simulink model "sampleModel372"  (R2021b)
settings: Solver=VariableStepAuto  StartTime=0.0  StopTime=10.0  RelTol=1e-3
undefined symbols (not defined in the file or in its folder): DiscIntNeverNeededParam, Newton, Raphson
libraries: simulink x10, slpidlib x1
settings Model: Creator=user  LastModifiedBy=user

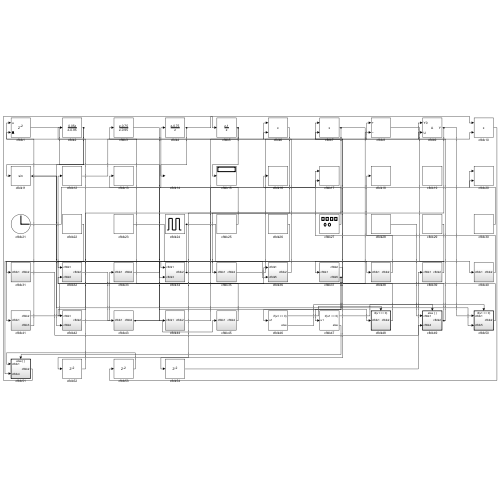
[thumbnail: Simulink's stored preview of the top-level diagram]
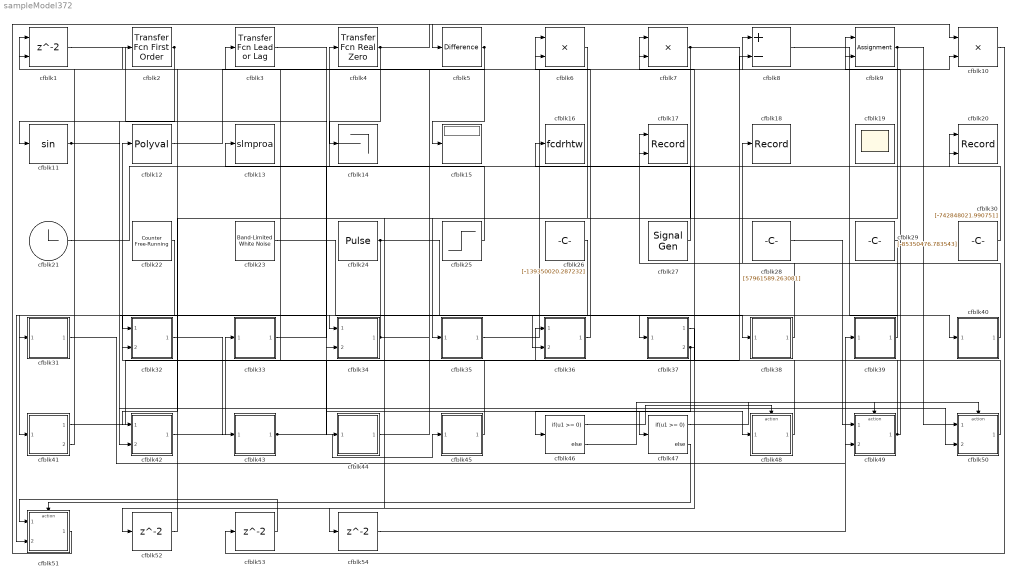
== system sampleModel372 ==
  cfblk1 : Delay  ShowEnablePort=on  SampleTime=1
      settings: InputPortMap=u0,e6
  cfblk10 : Product
  cfblk11 : Trigonometry
  cfblk12 : Polyval  Coefs=[ +2.081618890e-019, -1.441693666e-014, +4.719686976e-010, -8.536869453e-006, +1.621573104e-001, -8.087801117e+001 ]
  cfblk13 : ToWorkspace  VariableName=slmproa  SaveFormat=Timeseries  SampleTime=-1
  cfblk14 : Terminator
  cfblk15 : Display
  cfblk16 : ToWorkspace  VariableName=fcdrhtw  SaveFormat=Timeseries  SampleTime=-1
  cfblk17 : Record  FileSettingsInternal="{\"entries\":[{\"content\":{\"excelSettings\":{\"content\":{},\"type\":\"Streamout.ExcelSettings\"}},\"type\":\"Streamout.FileSettingStorage\",\"uuid\":\"b72ebad9-7056-485c-ac51-affa3a1e9353\"}],\"packageUris\":[\"http://schema.mathworks.com/mf0/streamout_blocks/R2020a\"],\"version\":\"1.0\"}"  Layout=[1 1]  SignalsInternal="{\"entries\":[{\"content\":{\"signals\":[{\"content\":{\"blockPath\":[\"sampleModel372/cfblk17\"],\"channel\":[],\"dimensions\":[1],\"domain\":\"sampleModel372/cfblk17\",\"lineColor\":\"#a2142f\",\"plots\":[1],\"port\":1,\"sid\":[\"\"],\"signalID\":15476,\"signalName\":\"cfblk44\"},\"type\":\"RecordBlkView.Signal\",\"uuid\":\"5dfffff1-d32b-4c9b-bc7a-56c91156797a\"},{\"content\":{\"blockPath\":[\"sampleModel372/cfblk17\"],\"channel\":[],\"dimensions\":[1],\"domain\":\"sampleModel372/cfblk17\",\"lineColor\":\"#139fff\",\"plots\":[1],\"port\":2,\"sid\":[\"\"],\"signalID\":15480,\"signalName\":\"cfblk38\"},\"type\":\"RecordBlkView.Signal\",\"uuid\":\"1c828c9b-06c4-4cee-a281-7d6f80fdea4d\"}]},\"type\":\"RecordBlkView.InputSignals\",\"uuid\":\"3665fb33-e0ad-4ba6-b3fb-c5c2c897735a\"}],\"packageUris\":[\"http://schema.mathworks.com/mf0/streamout_blocks/R2020a\"],\"version\":\"1.0\"}"  VisualizationBindings="{\"xyplotplugin\":{\"info\":[{\"series\":[{\"bindingParametersList\":[{\"parameter\":\"X-Axis\",\"signalID\":15476,\"signalName\":\"cfblk44\"},{\"parameter\":\"Y-Axis\",\"signalID\":15480,\"signalName\":\"cfblk38\"}],\"seriesID\":33208}],\"subplotID\":1}]}}"  CompatibilityTag=XY
  cfblk18 : Record  FileSettingsInternal="{\"entries\":[{\"content\":{\"excelSettings\":{\"content\":{},\"type\":\"Streamout.ExcelSettings\"}},\"type\":\"Streamout.FileSettingStorage\",\"uuid\":\"4903c734-b3f9-41ef-b0a2-174ee0824f37\"}],\"packageUris\":[\"http://schema.mathworks.com/mf0/streamout_blocks/R2020a\"],\"version\":\"1.0\"}"  SignalsInternal="{\"entries\":[{\"content\":{\"signals\":[{\"content\":{\"blockPath\":[\"sampleModel372/cfblk18\"],\"channel\":[],\"dimensions\":[1],\"domain\":\"sampleModel372/cfblk18\",\"lineColor\":\"#139fff\",\"plots\":[1],\"port\":1,\"sid\":[\"\"],\"signalID\":15484,\"signalName\":\"cfblk40\"},\"type\":\"RecordBlkView.Signal\",\"uuid\":\"409c68b6-5e7e-4f45-9345-40e6c37d40ec\"}]},\"type\":\"RecordBlkView.InputSignals\",\"uuid\":\"2f5d807f-9e3a-4e8f-8a79-911276b8b2d7\"}],\"packageUris\":[\"http://schema.mathworks.com/mf0/streamout_blocks/R2020a\"],\"version\":\"1.0\"}"  VisualizationBindings="{\"sparklinesplugin\":{\"info\":[{\"bindingParametersList\":[],\"subplotID\":1}]}}"
  cfblk19 : Scope
      settings: Floating=on
  cfblk2 : simulink/Discrete/Transfer Fcn First Order  PoleZ=0.95  ICPrevOutput=0.0  DoSatur=off
  cfblk20 : Record  FileSettingsInternal="{\"entries\":[{\"content\":{\"excelSettings\":{\"content\":{},\"type\":\"Streamout.ExcelSettings\"}},\"type\":\"Streamout.FileSettingStorage\",\"uuid\":\"bf4a5471-e929-4e71-bb99-9183bb1d84e0\"}],\"packageUris\":[\"http://schema.mathworks.com/mf0/streamout_blocks/R2020a\"],\"version\":\"1.0\"}"  Layout=[1 1]  SignalsInternal="{\"entries\":[{\"content\":{\"signals\":[{\"content\":{\"blockPath\":[\"sampleModel372/cfblk20\"],\"channel\":[],\"dimensions\":[1],\"domain\":\"sampleModel372/cfblk20\",\"lineColor\":\"#a2142f\",\"plots\":[1],\"port\":1,\"sid\":[\"\"],\"signalID\":15488,\"signalName\":\"cfblk33\"},\"type\":\"RecordBlkView.Signal\",\"uuid\":\"8512df04-6121-435b-9967-1d101e83269f\"},{\"content\":{\"blockPath\":[\"sampleModel372/cfblk20\"],\"channel\":[],\"dimensions\":[1],\"domain\":\"sampleModel372/cfblk20\",\"lineColor\":\"#139fff\",\"plots\":[1],\"port\":2,\"sid\":[\"\"],\"signalID\":15492,\"signalName\":\"cfblk30\"},\"type\":\"RecordBlkView.Signal\",\"uuid\":\"2aaa770d-525c-4c22-91f0-bfea3dd1c119\"}]},\"type\":\"RecordBlkView.InputSignals\",\"uuid\":\"b4e04a43-241c-40c6-8415-553e41d5351d\"}],\"packageUris\":[\"http://schema.mathworks.com/mf0/streamout_blocks/R2020a\"],\"version\":\"1.0\"}"  VisualizationBindings="{\"xyplotplugin\":{\"info\":[{\"series\":[{\"bindingParametersList\":[{\"parameter\":\"X-Axis\",\"signalID\":15488,\"signalName\":\"cfblk33\"},{\"parameter\":\"Y-Axis\",\"signalID\":15492,\"signalName\":\"cfblk30\"}],\"seriesID\":31222}],\"subplotID\":1}]}}"  CompatibilityTag=XY
  cfblk21 : Clock
  cfblk22 : simulink/Sources/Counter Free-Running  NumBits=[31.000000]  tsamp=-1
  cfblk23 : simulink/Sources/Band-Limited White Noise  Cov=[6149014609.811703]  Ts=0.1  seed=[2691800699.000000]
  cfblk24 : DiscretePulseGenerator  PulseType=Time based  Amplitude=[651098866.596543]  Period=[5211290.232713]  PulseWidth=5  PhaseDelay=[5.000000]
  cfblk25 : Step  Time=[32.000000]  Before=[-358467154.042758]  After=[548541878.025109]  SampleTime=0
  cfblk26 : Constant  Value=[-139350020.287232]  SampleTime=1
  cfblk27 : SignalGenerator  WaveForm=sawtooth  Amplitude=[-88090145.710845]
  cfblk28 : Constant  Value=[57961589.263081]  SampleTime=1
  cfblk29 : Constant  Value=[-85350476.783543]  SampleTime=1
  cfblk3 : simulink/Discrete/Transfer Fcn Lead or Lag  PoleZ=0.95  ZeroZ=0.75  ICPrevOutput=0.0  ICPrevInput=0.0  DoSatur=off
      settings: SourceProductBaseCode=SL
  cfblk30 : Constant  Value=[-742848021.990751]  SampleTime=1
  cfblk31 : Subsystem
  cfblk32 : Subsystem
  cfblk33 : Subsystem
  cfblk34 : Subsystem
  cfblk35 : Subsystem
  cfblk36 : Subsystem
  cfblk37 : Subsystem
  cfblk38 : Subsystem
  cfblk39 : Subsystem
  cfblk4 : simulink/Discrete/Transfer Fcn Real Zero  ZeroZ=0.75  ICPrevInput=0.0  DoSatur=off
      settings: SourceProductBaseCode=SL
  cfblk40 : Subsystem
  cfblk41 : Subsystem
  cfblk42 : Subsystem
  cfblk43 : Subsystem
  cfblk44 : Subsystem
  cfblk45 : Subsystem
  cfblk46 : If  IfExpression=u1 >= 0  SampleTime=1
  cfblk47 : If  IfExpression=u1 >= 0  SampleTime=1
  cfblk48 : Subsystem  TreatAsAtomicUnit=on
  cfblk49 : Subsystem  TreatAsAtomicUnit=on
  cfblk5 : simulink/Discrete/Difference  ICPrevInput=0.0  OutMin=[]  OutMax=[]  OutDataTypeStr=Inherit: Inherit via back propagation  OutDataType=fixdt(1, 16)  OutScaling=2^-10  DoSatur=off
  cfblk50 : Subsystem  TreatAsAtomicUnit=on
  cfblk51 : Subsystem  TreatAsAtomicUnit=on
  cfblk52 : Delay  SampleTime=1
  cfblk53 : Delay  SampleTime=1
  cfblk54 : Delay  SampleTime=1
  cfblk6 : Product  Inputs=**
  cfblk7 : Product
  cfblk8 : Sum  Inputs=+-
  cfblk9 : Assignment  DiagnosticForDimensions=Warning  IndexOptions=Index vector (dialog)  Indices=1  OutputSizes=1
  wires:
  cfblk9/1 -> cfblk35/1(cfblk1), cfblk50/1(cfblk1)
  cfblk35/1(cfblk2) -> cfblk8/1
  cfblk21/1 -> cfblk4/1
  cfblk5/1 -> cfblk15/1, cfblk1/2
  cfblk25/1 -> cfblk13/1
  cfblk3/1 -> cfblk48/1(cfblk1)
  cfblk43/1(cfblk2) -> cfblk45/1(cfblk1), cfblk36/1(cfblk1)
  cfblk4/1 -> cfblk14/1, cfblk10/1
  cfblk45/1(cfblk2) -> cfblk12/1
  cfblk2/1 -> cfblk11/1, cfblk42/2(cfblk4)
  cfblk31/1(cfblk2) -> cfblk39/1(cfblk1)
  cfblk42/1(cfblk2) -> cfblk33/1(cfblk1)
  cfblk26/1 -> cfblk34/1(cfblk1)
  cfblk51/1(cfblk2) -> cfblk5/1
  cfblk33/1(cfblk2) -> cfblk20/1
  cfblk50/1(cfblk2) -> cfblk3/1
  cfblk29/1 -> cfblk32/1(cfblk1)
  cfblk22/1 -> cfblk41/1(cfblk1)
  cfblk30/1 -> cfblk20/2
  cfblk1/1 -> cfblk44/1(cfblk1)
  cfblk39/1(cfblk2) -> cfblk37/1(cfblk1)
  cfblk28/1 -> cfblk49/1(cfblk1)
  cfblk27/1 -> cfblk16/1
  cfblk12/1 -> cfblk9/1
  cfblk24/1 -> cfblk51/2(cfblk4), cfblk36/2(cfblk5)
  cfblk36/1(cfblk2) -> cfblk6/1
  cfblk44/1(cfblk2) -> cfblk17/1
  cfblk40/1(cfblk2) -> cfblk18/1
  cfblk38/1(cfblk2) -> cfblk17/2
  cfblk8/1 -> cfblk40/1(cfblk1)
  cfblk23/1 -> cfblk38/1(cfblk1)
  cfblk11/1 -> cfblk34/2(cfblk3), cfblk50/2(cfblk5)
  cfblk41/1(cfblk2) -> cfblk8/2
  cfblk37/2(cfblk5) -> cfblk47/1, cfblk7/2, cfblk46/1
  cfblk48/1(cfblk2) -> cfblk7/1
  cfblk32/1(cfblk2) -> cfblk43/1(cfblk1)
  cfblk41/2(cfblk3) -> cfblk1/1
  cfblk49/1(cfblk2) -> cfblk9/2, cfblk32/2(cfblk3)
  cfblk7/1 -> cfblk42/1(cfblk1), cfblk10/2
  cfblk34/1(cfblk2) -> cfblk31/1(cfblk1), cfblk6/2
  cfblk46/1 -> cfblk48/Action
  cfblk46/2 -> cfblk49/Action
  cfblk47/1 -> cfblk50/Action
  cfblk47/2 -> cfblk51/Action
  cfblk37/1(cfblk2) -> cfblk52/1
  cfblk52/1 -> cfblk2/1
  cfblk10/1 -> cfblk53/1
  cfblk53/1 -> cfblk51/1(cfblk1)
  cfblk6/1 -> cfblk54/1
  cfblk54/1 -> cfblk49/2(cfblk4)

== system sampleModel372/cfblk31 ==
  cfblk1 : Inport
  cfblk3 : slpidlib/PID Controller (2DOF)  Controller=PID  Form=Parallel  TimeDomain=Discrete-time  UseExternalTs=off  SampleTime=1  IntegratorMethod=Forward Euler  FilterMethod=Forward Euler  ControllerParametersSource=internal  P=1  I=1  D=0  UseFilter=on  N=100  b=1  c=1  TunerSelectOption=Transfer Function Based (PID Tuner App)  InitialConditionSource=internal  InitialConditionForIntegrator=0  InitialConditionForFilter=0  DifferentiatorICPrevScaledInput=0  ExternalReset=none  TrackingMode=off  Kt=1  LimitOutput=off  SatLimitsSource=internal  UpperSaturationLimit=inf  LowerSaturationLimit=-inf  LinearizeAsGain=off  AntiWindupMode=none  Kb=1  POutMin=[]  POutMax=[]  IOutMin=[]  IOutMax=[]  DOutMin=[]  DOutMax=[]  NOutMin=[]  NOutMax=[]  bOutMin=[]  bOutMax=[]  cOutMin=[]  cOutMax=[]  SumOutMin=[]  SumOutMax=[]  SaturationOutMin=[]  SaturationOutMax=[]  PParamMin=[]  PParamMax=[]  IParamMin=[]  IParamMax=[]  DParamMin=[]  DParamMax=[]  NParamMin=[]  NParamMax=[]  bParamMin=[]  bParamMax=[]  cParamMin=[]  cParamMax=[]  KbParamMin=[]  KbParamMax=[]  KtParamMin=[]  KtParamMax=[]  KbOutMin=[]  KbOutMax=[]  KtOutMin=[]  KtOutMax=[]  IntegratorOutMin=[]  IntegratorOutMax=[]  FilterOutMin=[]  FilterOutMax=[]  SumI1OutMin=[]  SumI1OutMax=[]  SumI2OutMin=[]  SumI2OutMax=[]  SumI3OutMin=[]  SumI3OutMax=[]  SumI4OutMin=[]  SumI4OutMax=[]  SumDOutMin=[]  SumDOutMax=[]  Sum1OutMin=[]  Sum1OutMax=[]  Sum2OutMin=[]  Sum2OutMax=[]  Sum3OutMin=[]  Sum3OutMax=[]  DifferentiatorOutMin=[]  DifferentiatorOutMax=[]  FilterDiffOutCoefMin=[]  FilterDiffOutCoefMax=[]  ReciprocalOutMin=[]  ReciprocalOutMax=[]  SumDenOutMin=[]  SumDenOutMax=[]  SumNumOutMin=[]  SumNumOutMax=[]  DivideOutMin=[]  DivideOutMax=[]  UdiffTsProdOutMin=[]  UdiffTsProdOutMax=[]  NTsProdOutMin=[]  NTsProdOutMax=[]  UintegralTsProdOutMin=[]  UintegralTsProdOutMax=[]  UngainTsProdOutMin=[]  UngainTsProdOutMax=[]  IntegratorContinuousStateAttributes=''  IntegratorStateMustResolveToSignalObject=off  IntegratorRTWStateStorageClass=Auto  FilterContinuousStateAttributes=''  FilterStateMustResolveToSignalObject=off  FilterRTWStateStorageClass=Auto  ParallelPVariant=InternalParameters  IdealPVariant=Disabled  IVariant=InternalParameters  DVariant=InternalParameters  bVariant=InternalParameters  cVariant=InternalParameters  IntegratorVariant=Discrete  SatVariant=Disabled  AWVariant=Passthrough  PCopyVariant=Disabled  TRVariant=Disabled  FdbkBlocksVariant=Forward  IdealPFdbkVariant=Disabled  SatFdbkVariant=Disabled  DerivativeFilterVariant=ForwardEulerFilter  NVariant=InternalParameters  NCopyVariant=Disabled  FilterICVariant=InternalICsFilter  IntegratorICVariant=InternalICs  ExternalResetVariant=Disabled  TRSumVariant=Passthrough  SumFdbkVariant=Disabled  SumVariant=Sum_PID  TsampFilterVariant=InternalTs  TsampNgainVariant=Passthrough  TsampIntegralVariant=Passthrough  ExternalSaturationOutDataTypeStr=Inherit: Same as second input
      settings: SourceProductBaseCode=SL
  cfblk2 : Outport
  wires:
  cfblk3/1 -> cfblk2/1
  cfblk1/1 -> cfblk3/1, cfblk3/2

== system sampleModel372/cfblk32 ==
  cfblk1 : Inport
  cfblk3 : Inport  Port=2
  cfblk2 : Outport
  wires:
  cfblk3/1 -> cfblk2/1

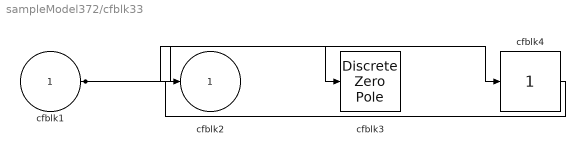
== system sampleModel372/cfblk33 ==
  cfblk1 : Inport
  cfblk3 : DiscreteZeroPole  Poles=[0 0.5]  Gain=1
  cfblk4 : simulink/Math Operations/Slider Gain  gain=1  low=0  high=2
  cfblk2 : Outport
  wires:
  cfblk1/1 -> cfblk4/1, cfblk3/1
  cfblk4/1 -> cfblk2/1

== system sampleModel372/cfblk34 ==
  cfblk1 : Inport
  cfblk3 : Inport  Port=2
  cfblk2 : Outport
  wires:
  cfblk1/1 -> cfblk2/1

== system sampleModel372/cfblk35 ==
  cfblk1 : Inport
  cfblk3 : Gain  Gain=[-728602768.231833]
  cfblk2 : Outport
  wires:
  cfblk3/1 -> cfblk2/1
  cfblk1/1 -> cfblk3/1

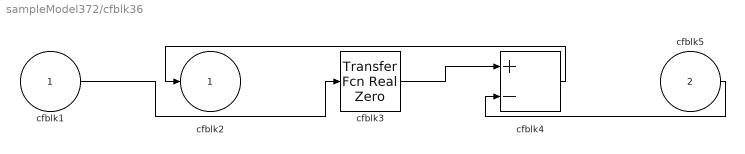
== system sampleModel372/cfblk36 ==
  cfblk1 : Inport
  cfblk5 : Inport  Port=2
  cfblk3 : simulink/Discrete/Transfer Fcn Real Zero  ZeroZ=0.75  ICPrevInput=0.0  DoSatur=off
      settings: SourceProductBaseCode=SL
  cfblk4 : Sum  Inputs=+-
  cfblk2 : Outport
  wires:
  cfblk4/1 -> cfblk2/1
  cfblk3/1 -> cfblk4/1
  cfblk5/1 -> cfblk4/2
  cfblk1/1 -> cfblk3/1

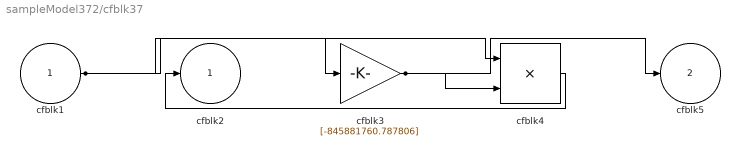
== system sampleModel372/cfblk37 ==
  cfblk1 : Inport
  cfblk3 : Gain  Gain=[-845881760.787806]
  cfblk4 : Product
  cfblk2 : Outport
  cfblk5 : Outport  Port=2
  wires:
  cfblk3/1 -> cfblk5/1, cfblk4/2
  cfblk4/1 -> cfblk2/1
  cfblk1/1 -> cfblk3/1, cfblk4/1

== system sampleModel372/cfblk38 ==
  cfblk1 : Inport
  cfblk3 : Signum
  cfblk2 : Outport
  wires:
  cfblk3/1 -> cfblk2/1
  cfblk1/1 -> cfblk3/1

== system sampleModel372/cfblk39 ==
  cfblk1 : Inport
  cfblk3 : DiscreteTransferFcn  SampleTime=1
  cfblk2 : Outport
  wires:
  cfblk1/1 -> cfblk3/1
  cfblk3/1 -> cfblk2/1

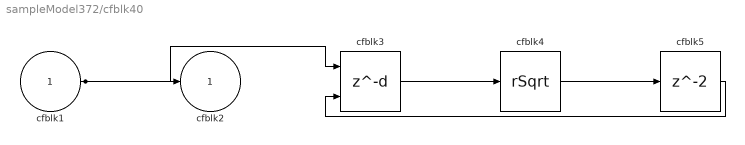
== system sampleModel372/cfblk40 ==
  cfblk1 : Inport
  cfblk3 : Delay  DelayLengthSource=Input port  SampleTime=1
      settings: InputPortMap=u0,p1
  cfblk4 : Sqrt  Operator=rSqrt  AlgorithmType=Newton-Raphson  SaturateOnIntegerOverflow=on
  cfblk5 : Delay  SampleTime=1
  cfblk2 : Outport
  wires:
  cfblk3/1 -> cfblk4/1
  cfblk1/1 -> cfblk3/1, cfblk2/1
  cfblk4/1 -> cfblk5/1
  cfblk5/1 -> cfblk3/2

== system sampleModel372/cfblk41 ==
  cfblk1 : Inport
  cfblk2 : Outport
  cfblk3 : Outport  Port=2
  wires:
  cfblk1/1 -> cfblk2/1, cfblk3/1

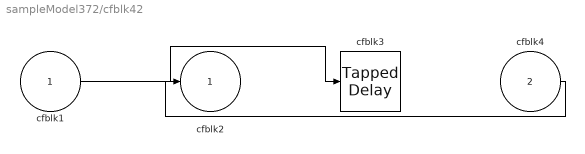
== system sampleModel372/cfblk42 ==
  cfblk1 : Inport
  cfblk4 : Inport  Port=2
  cfblk3 : simulink/Discrete/Tapped Delay  vinit=0.0  samptime=-1  NumDelays=1  DelayOrder=Oldest  includeCurrent=off
  cfblk2 : Outport
  wires:
  cfblk1/1 -> cfblk3/1
  cfblk4/1 -> cfblk2/1

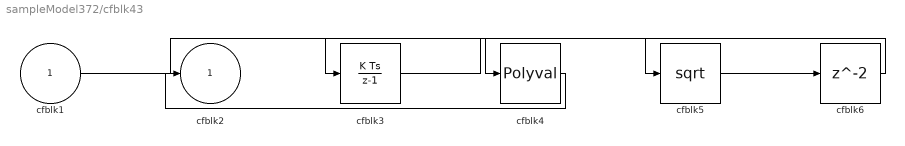
== system sampleModel372/cfblk43 ==
  cfblk1 : Inport
  cfblk3 : DiscreteIntegrator  ICPrevOutput=DiscIntNeverNeededParam  ICPrevScaledInput=DiscIntNeverNeededParam
  cfblk4 : Polyval  Coefs=[ +2.081618890e-019, -1.441693666e-014, +4.719686976e-010, -8.536869453e-006, +1.621573104e-001, -8.087801117e+001 ]
  cfblk5 : Sqrt  SaturateOnIntegerOverflow=on
  cfblk6 : Delay  SampleTime=1
  cfblk2 : Outport
  wires:
  cfblk1/1 -> cfblk4/1
  cfblk4/1 -> cfblk2/1
  cfblk3/1 -> cfblk5/1
  cfblk5/1 -> cfblk6/1
  cfblk6/1 -> cfblk3/1

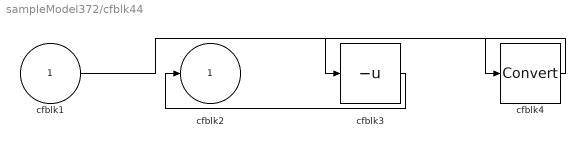
== system sampleModel372/cfblk44 ==
  cfblk1 : Inport
  cfblk3 : UnaryMinus
  cfblk4 : DataTypeConversion
  cfblk2 : Outport
  wires:
  cfblk3/1 -> cfblk2/1
  cfblk1/1 -> cfblk4/1
  cfblk4/1 -> cfblk3/1

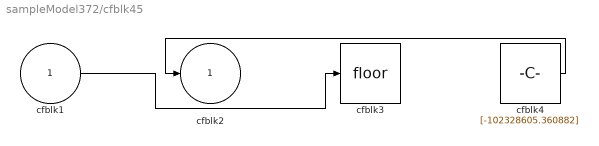
== system sampleModel372/cfblk45 ==
  cfblk1 : Inport
  cfblk3 : Rounding
  cfblk4 : Constant  Value=[-102328605.360882]  SampleTime=1
  cfblk2 : Outport
  wires:
  cfblk4/1 -> cfblk2/1
  cfblk1/1 -> cfblk3/1

== system sampleModel372/cfblk48 ==
  cfblk1 : Inport
  Action Port : ActionPort  ActionPortLabel=if(u1 >= 0)
  cfblk3 : Bias  Bias=[-32648959.725881]
  cfblk2 : Outport
  wires:
  cfblk1/1 -> cfblk3/1
  cfblk3/1 -> cfblk2/1

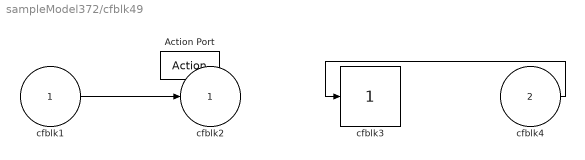
== system sampleModel372/cfblk49 ==
  cfblk1 : Inport
  cfblk4 : Inport  Port=2
  Action Port : ActionPort  ActionPortLabel=else
  cfblk3 : simulink/Math Operations/Slider Gain  gain=1  low=0  high=2
  cfblk2 : Outport
  wires:
  cfblk4/1 -> cfblk3/1
  cfblk1/1 -> cfblk2/1

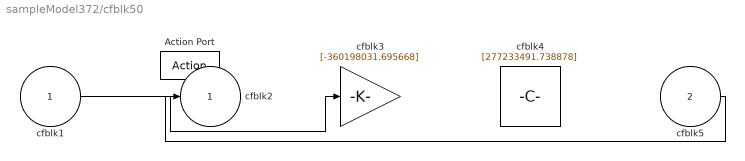
== system sampleModel372/cfblk50 ==
  cfblk1 : Inport
  cfblk5 : Inport  Port=2
  Action Port : ActionPort  ActionPortLabel=if(u1 >= 0)
  cfblk3 : Gain  Gain=[-360198031.695668]
  cfblk4 : Constant  Value=[277233491.738878]  SampleTime=1
  cfblk2 : Outport
  wires:
  cfblk1/1 -> cfblk3/1
  cfblk5/1 -> cfblk2/1

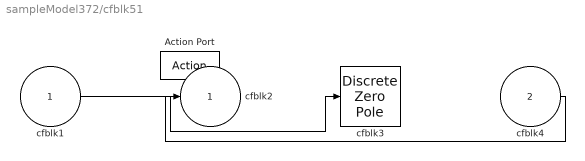
== system sampleModel372/cfblk51 ==
  cfblk1 : Inport
  cfblk4 : Inport  Port=2
  Action Port : ActionPort  ActionPortLabel=else
  cfblk3 : DiscreteZeroPole  Poles=[0 0.5]  Gain=1  SampleTime=-1
  cfblk2 : Outport
  wires:
  cfblk1/1 -> cfblk3/1
  cfblk4/1 -> cfblk2/1
